simulink model "bb_lqr_hg_sl"  (Simulink 7.9)
settings: Solver=FixedStepDiscrete  StartTime=0.0  StopTime=inf  FixedStep=ts  RelTol=1e-3
values from neighbouring files (symbols this model uses):
  F = lqr(Pbb,Q,R)    [bb_lqr_hg.m]    (also in bb_lqr_servo_hg.m = Ftmp(:,1:4))
  r1 = 20    [bb_lqr_hg.m]    (also in bb_lqr_servo_hg.m = 15; bb_pid_hg.m = 15; bb_pid_rc.m = 15)
  ts = 0.02    [sim_param.mat]
undefined symbols (not defined in the file or in its folder): denlpf, numlpf
libraries: arduino_io_lib x6, simulink x2
settings Model: Creator=hirata  LastModifiedBy=hirata
settings DebuggingCC: FcnCallInpInsideContextMsg=Use local settings
settings GRTTargetCC: CombineOutputUpdateFcns=off  GRTInterface=on

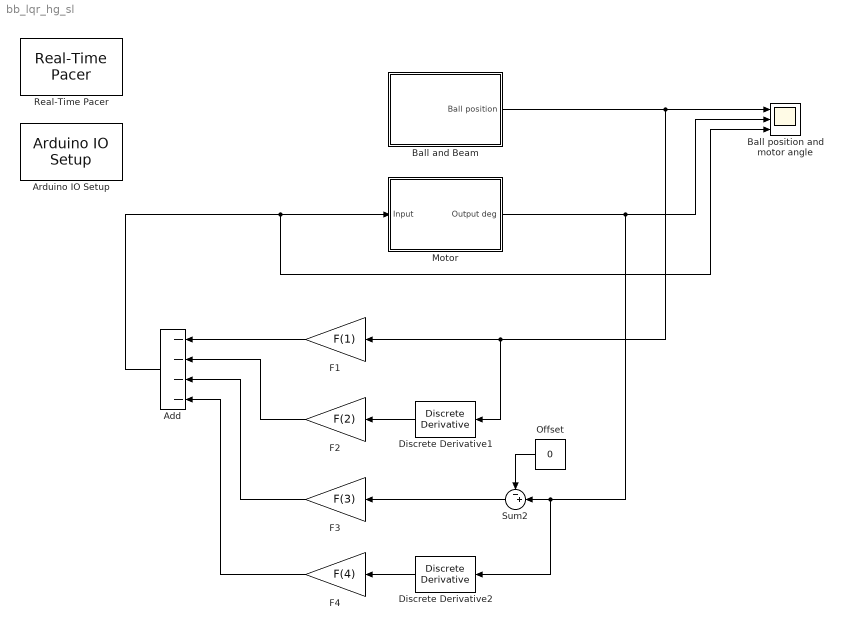
== system bb_lqr_hg_sl ==
  Add : Sum  Inputs=----
  Arduino IO Setup : arduino_io_lib/Arduino IO Setup  Priority=3  arduinoVar=Temporary arduino variable: Arduino1  workspaceVarName=a  comPort=COM3
  Ball and Beam : Subsystem
  Ball position and motor angle : Scope  NumInputPorts=3
      settings: TimeRange=30  YMin=-15~-50~-5  YMax=25~50~5
  Discrete Derivative1 : simulink/Discrete/Discrete Derivative  gainval=1.0  ICPrevScaledInput=0.0  InputProcessing=Inherited  OutMin=[]  OutMax=[]  OutDataType=fixdt(1, 16)  OutScaling=2^-10  DoSatur=off
  Discrete Derivative2 : simulink/Discrete/Discrete Derivative  gainval=1.0  ICPrevScaledInput=0.0  InputProcessing=Inherited  OutMin=[]  OutMax=[]  OutDataType=fixdt(1, 16)  OutScaling=2^-10  DoSatur=off
  F1 : Gain  Gain=F(1)
  F2 : Gain  Gain=F(2)
  F3 : Gain  Gain=F(3)
  F4 : Gain  Gain=F(4)
  Motor : Subsystem
  Offset : Constant  Value=0  SampleTime=ts
  Real-Time Pacer : arduino_io_lib/Real-Time Pacer  simTimePerRealTime=1
  Sum2 : Sum  Inputs=-+|
  wires:
  Discrete Derivative1/1 -> F2/1
  Discrete Derivative2/1 -> F4/1
  Ball and Beam/1(Ball position) -> Discrete Derivative1/1, F1/1, Ball position and motor angle/1
  Motor/1(Output deg) -> Sum2/2, Discrete Derivative2/1, Ball position and motor angle/2
  F1/1 -> Add/1
  F2/1 -> Add/2
  F4/1 -> Add/4
  F3/1 -> Add/3
  Add/1 -> Motor/1(Input), Ball position and motor angle/3
  Sum2/1 -> F3/1
  Offset/1 -> Sum2/1

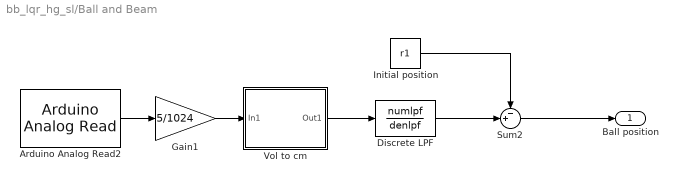
== system bb_lqr_hg_sl/Ball and Beam ==
  Arduino Analog Read2 : arduino_io_lib/Arduino Analog Read  arduinoVar=Temporary arduino variable: Arduino1  arduinoPin=2  T=ts
  Discrete LPF : DiscreteTransferFcn  Numerator=numlpf  Denominator=denlpf
  Gain1 : Gain  Gain=5/1024
  Initial position : Constant  Value=r1
  Sum2 : Sum  Inputs=-+|
  Vol to cm : Subsystem
  Ball position : Outport
  wires:
  Arduino Analog Read2/1 -> Gain1/1
  Gain1/1 -> Vol to cm/1(In1)
  Vol to cm/1(Out1) -> Discrete LPF/1
  Initial position/1 -> Sum2/1
  Discrete LPF/1 -> Sum2/2
  Sum2/1 -> Ball position/1

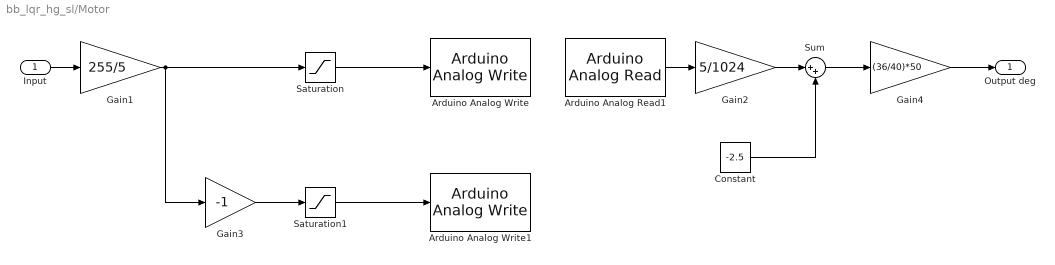
== system bb_lqr_hg_sl/Motor ==
  Input : Inport
  Arduino Analog Read1 : arduino_io_lib/Arduino Analog Read  arduinoVar=Temporary arduino variable: Arduino1  arduinoPin=0  T=ts
  Arduino Analog Write : arduino_io_lib/Arduino Analog Write  arduinoVar=Temporary arduino variable: Arduino1  arduinoPin=3  T=ts
  Arduino Analog Write1 : arduino_io_lib/Arduino Analog Write  arduinoVar=Temporary arduino variable: Arduino1  arduinoPin=5  T=ts
  Constant : Constant  Value=-2.5
  Gain1 : Gain  Gain=255/5
  Gain2 : Gain  Gain=5/1024
  Gain3 : Gain  Gain=-1
  Gain4 : Gain  Gain=(36/40)*50
  Saturation : Saturate  UpperLimit=255  LowerLimit=0
  Saturation1 : Saturate  UpperLimit=255  LowerLimit=0
  Sum : Sum  Inputs=|++
  Output deg : Outport
  wires:
  Input/1 -> Gain1/1
  Arduino Analog Read1/1 -> Gain2/1
  Saturation/1 -> Arduino Analog Write/1
  Gain1/1 -> Gain3/1, Saturation/1
  Saturation1/1 -> Arduino Analog Write1/1
  Gain4/1 -> Output deg/1
  Gain2/1 -> Sum/1
  Sum/1 -> Gain4/1
  Constant/1 -> Sum/2
  Gain3/1 -> Saturation1/1

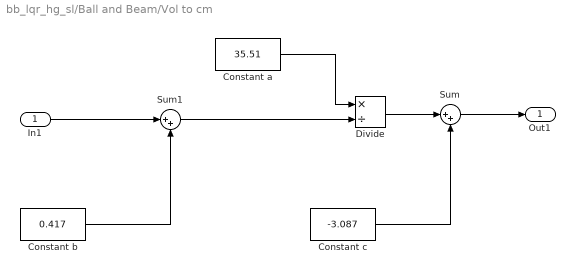
== system bb_lqr_hg_sl/Ball and Beam/Vol to cm ==
  In1 : Inport
  Constant a : Constant  Value=35.51
  Constant b : Constant  Value=0.417
  Constant c : Constant  Value=-3.087
  Divide : Product  Inputs=*/
  Sum : Sum  Inputs=|++
  Sum1 : Sum  Inputs=|++
  Out1 : Outport
  wires:
  Constant a/1 -> Divide/1
  Divide/1 -> Sum/1
  Sum/1 -> Out1/1
  Constant c/1 -> Sum/2
  In1/1 -> Sum1/1
  Sum1/1 -> Divide/2
  Constant b/1 -> Sum1/2
